simulink model "motorsim_PWM"  (R2021a)
settings: Solver=VariableStepAuto  StartTime=0.0  StopTime=10.0  RelTol=1e-3
values from neighbouring files (symbols this model uses):
  b = .5    (= 0.5)    [RunStep_response.m]    (also in Runmotorsim.m)
  J = .05    (= 0.05)    [RunStep_response.m]    (also in Runmotorsim.m)
  Ke = .5    (= 0.5)    [RunStep_response.m]    (also in Runmotorsim.m)
  Kt = 1    [RunStep_response.m]    (also in Runmotorsim.m = 0.5)
  Ra = 1    [RunStep_response.m]    (also in Runmotorsim.m)
libraries: simulink x2
settings Model: Creator=Beau Collins  LastModifiedBy=abcollins
settings SolverCC: AlgebraicLoopSolver=TrustRegion
settings DebuggingCC: SFMachineParentedDataDiag=warning

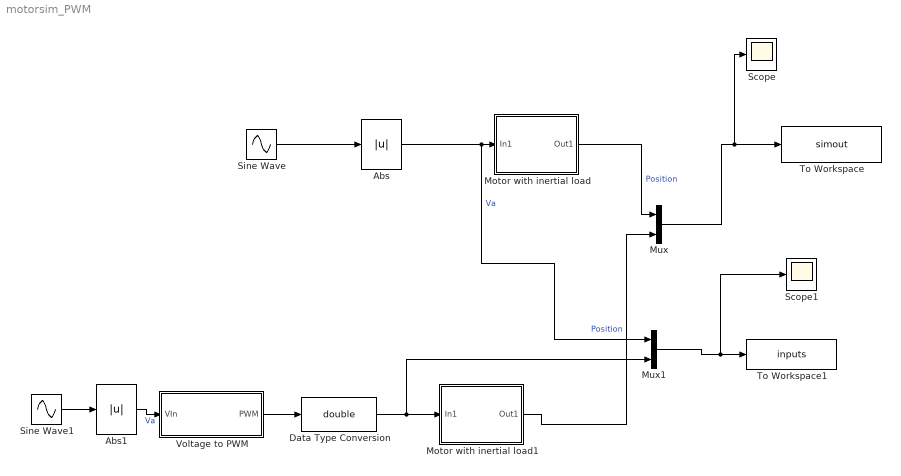
== system motorsim_PWM ==
  Abs : Abs
  Abs1 : Abs
  Data Type Conversion : DataTypeConversion  OutDataTypeStr=double
  Motor with inertial load : Subsystem
  Motor with inertial load1 : Subsystem
  Mux : Mux  Inputs=2
  Mux1 : Mux  Inputs=2
  Scope : Scope
  Scope1 : Scope
  Sine Wave : Sin  SampleTime=0
  Sine Wave1 : Sin  SampleTime=0
  To Workspace : ToWorkspace  VariableName=simout  SaveFormat=Timeseries  SampleTime=-1
  To Workspace1 : ToWorkspace  VariableName=inputs  SaveFormat=Timeseries  SampleTime=-1
  Voltage to PWM : Subsystem
  wires:
  Sine Wave/1 -> Abs/1
  Abs/1 -> Mux1/1, Motor with inertial load/1(In1)  "Va"
  Motor with inertial load/1(Out1) -> Mux/1  "Position"
  Sine Wave1/1 -> Abs1/1
  Abs1/1 -> Voltage to PWM/1(VIn)  "Va"
  Mux/1 -> Scope/1, To Workspace/1
  Mux1/1 -> Scope1/1, To Workspace1/1
  Motor with inertial load1/1(Out1) -> Mux/2  "Position"
  Voltage to PWM/1(PWM) -> Data Type Conversion/1
  Data Type Conversion/1 -> Mux1/2, Motor with inertial load1/1(In1)

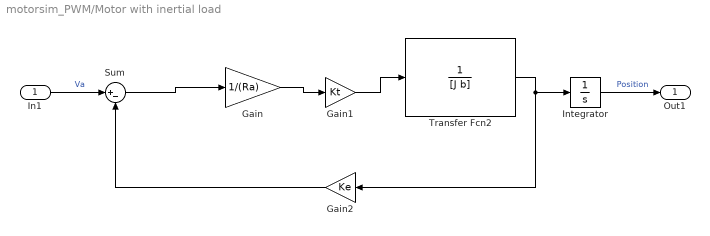
== system motorsim_PWM/Motor with inertial load ==
  In1 : Inport
  Gain : Gain  Gain=1/(Ra)
  Gain1 : Gain  Gain=Kt
  Gain2 : Gain  Gain=Ke
  Integrator : Integrator
  Sum : Sum  Inputs=|+-
  Transfer Fcn2 : TransferFcn  Denominator=[J b]  ContinuousStateAttributes='Transfer_Fcn'
  Out1 : Outport
  wires:
  In1/1 -> Sum/1  "Va"
  Transfer Fcn2/1 -> Gain2/1, Integrator/1
  Sum/1 -> Gain/1
  Gain2/1 -> Sum/2
  Gain/1 -> Gain1/1
  Integrator/1 -> Out1/1  "Position"
  Gain1/1 -> Transfer Fcn2/1

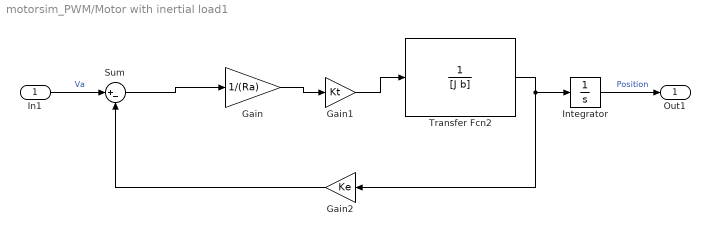
== system motorsim_PWM/Motor with inertial load1 ==
  In1 : Inport
  Gain : Gain  Gain=1/(Ra)
  Gain1 : Gain  Gain=Kt
  Gain2 : Gain  Gain=Ke
  Integrator : Integrator
  Sum : Sum  Inputs=|+-
  Transfer Fcn2 : TransferFcn  Denominator=[J b]  ContinuousStateAttributes='Transfer_Fcn'
  Out1 : Outport
  wires:
  In1/1 -> Sum/1  "Va"
  Transfer Fcn2/1 -> Gain2/1, Integrator/1
  Sum/1 -> Gain/1
  Gain2/1 -> Sum/2
  Gain/1 -> Gain1/1
  Integrator/1 -> Out1/1  "Position"
  Gain1/1 -> Transfer Fcn2/1

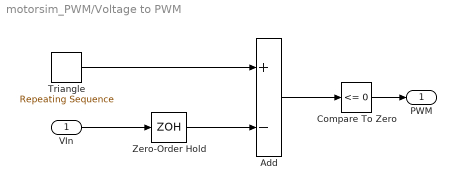
== system motorsim_PWM/Voltage to PWM ==
  VIn : Inport
  Add : Sum  Inputs=+-  SampleTime=1/10000
  Compare To Zero : simulink/Logic and Bit Operations/Compare To Zero  relop=<=  OutDataTypeStr=uint8
  Triangle : simulink/Sources/Repeating Sequence  rep_seq_t=[0 1/100/4 3/100/4 1/100]*25  rep_seq_y=[0.5 0 1 0.5]
  Zero-Order Hold : ZeroOrderHold  SampleTime=1/10000
  PWM : Outport  VectorParamsAs1DForOutWhenUnconnected=off
  wires:
  Triangle/1 -> Add/1
  VIn/1 -> Zero-Order Hold/1
  Add/1 -> Compare To Zero/1
  Compare To Zero/1 -> PWM/1
  Zero-Order Hold/1 -> Add/2
